simulink model "model1"  (R2021b)
settings: Solver=VariableStepAuto  StartTime=0.0  StopTime=10.0  RelTol=1e-3
values from neighbouring files (symbols this model uses):
  A_m = [     0      1 ... (first row only)    [config.m]
  b_m = [0 ... (first row only)    [config.m]
  C_m = C    [config.m]
settings Model: Creator=popov  LastModifiedBy=popov

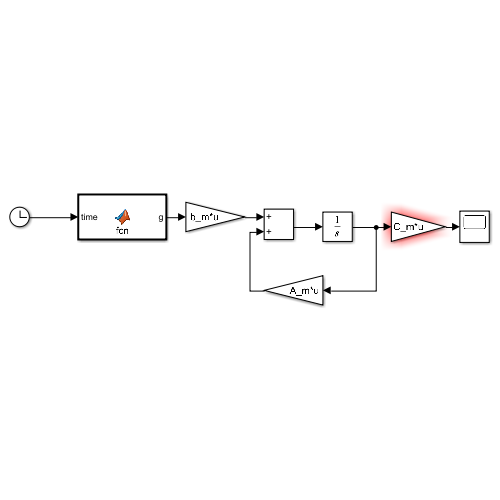
[thumbnail: Simulink's stored preview of the top-level diagram]
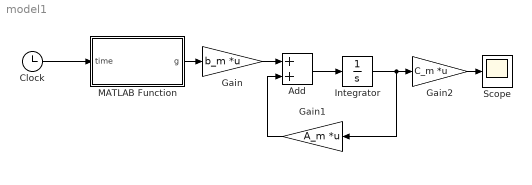
== system model1 ==
  Add : Sum
  Clock : Clock
  Gain : Gain  Gain=b_m  Multiplication=Matrix(K*u)
  Gain1 : Gain  Gain=A_m  Multiplication=Matrix(K*u)
  Gain2 : Gain  Gain=C_m  Multiplication=Matrix(K*u)
  Integrator : Integrator
  MATLAB Function : MATLAB Function  TreatAsAtomicUnit=on
  Scope : Scope
  wires:
  Clock/1 -> MATLAB Function/1(time)
  Gain/1 -> Add/1
  Add/1 -> Integrator/1
  Gain1/1 -> Add/2
  MATLAB Function/1(g) -> Gain/1
  Integrator/1 -> Gain1/1, Gain2/1
  Gain2/1 -> Scope/1

== matlab function model1/MATLAB Function ==
  data: time input; g output
function g = fcn(time)

g = 2*sign(sin(0.4*time)) + 3;
